simulink model "Simulink9"  (R2016b)
settings: Solver=ode4  StartTime=0.0  StopTime=30.0  FixedStep=0.005  RelTol=1e-3
values from neighbouring files (symbols this model uses):
  Kf = (1/tauf)    (= 20)    [Ejercicio9.m]
  Kt = 10/90    (= 0.111111111111)    [Ejercicio9.m]
  tauf = 1/wcf    (= 0.05)    [Ejercicio9.m]
  Vmax = 60    [Ejercicio9.m]
  wcf = 20    [Ejercicio9.m]
  wn = 20    [Ejercicio9.m]
  Xmax = 90    [Ejercicio9.m]
  zeta = 0.85    [Ejercicio9.m]
  zetaf = 1    [Ejercicio9.m]
undefined symbols (not defined in the file or in its folder): Tm
libraries: simulink x6
settings Model: Creator=elena  LastModifiedBy=elena
settings DataIOCC: ReturnWorkspaceOutputs=on
settings DebuggingCC: SFMachineParentedDataDiag=error
settings SFSimCC: SimUseLocalCustomCode=on
settings RTWCC: RTWUseLocalCustomCode=on

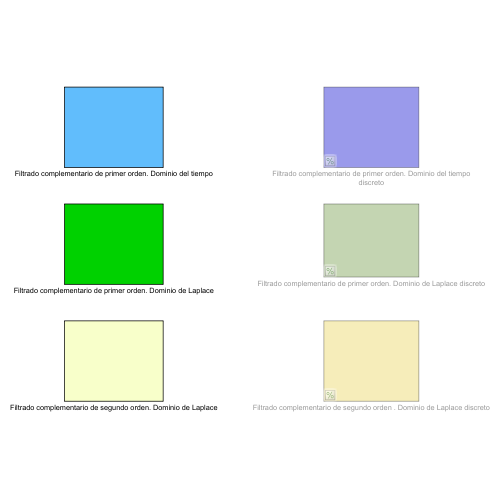
[thumbnail: Simulink's stored preview of the top-level diagram]
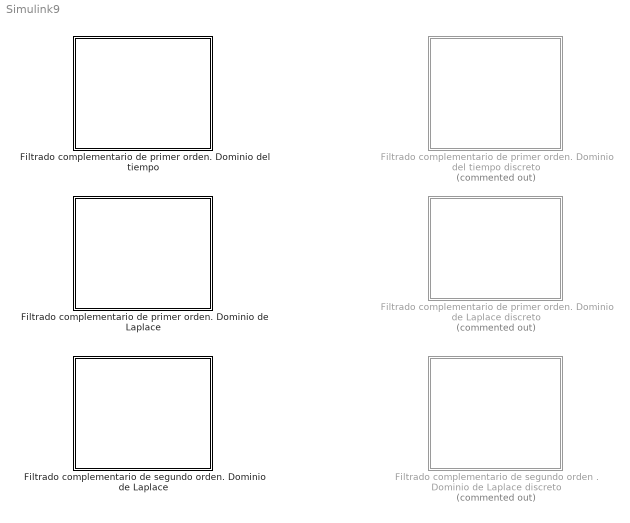
== system Simulink9 ==
  Filtrado complementario de primer orden. Dominio de Laplace : Subsystem
  Filtrado complementario de primer orden. Dominio de Laplace discreto : Subsystem  Commented=on
  "Filtrado complementario de primer orden. Dominio del tiempo " : Subsystem
  Filtrado complementario de primer orden. Dominio del tiempo discreto : Subsystem  Commented=on
  Filtrado complementario de segundo orden . Dominio de Laplace discreto : Subsystem  Commented=on
  Filtrado complementario de segundo orden. Dominio de Laplace : Subsystem

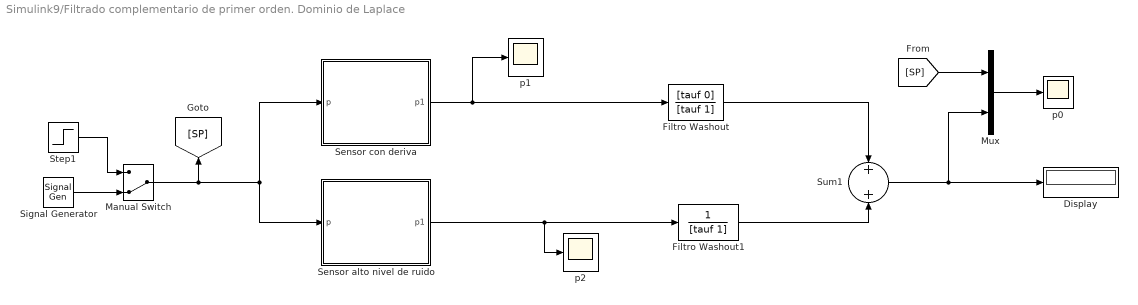
== system Simulink9/Filtrado complementario de primer orden. Dominio de Laplace ==
  Display : Display
  Filtro Washout : TransferFcn  Numerator=[tauf 0]  Denominator=[tauf 1]
  Filtro Washout1 : TransferFcn  Denominator=[tauf 1]
  Manual Switch : ManualSwitch  CurrentSetting=0
  Mux : Mux  Inputs=2
  Sensor alto nivel de ruido : Subsystem
  Sensor con deriva : Subsystem
  Signal Generator : SignalGenerator  Units=rad/sec
  Step1 : Step  SampleTime=0
  Sum1 : Sum
  p0 : Scope
  p1 : Scope
  p2 : Scope
  wires:
  Sensor alto nivel de ruido/1(p1) -> p2/1, Filtro Washout1/1
  Sensor con deriva/1(p1) -> p1/1, Filtro Washout/1
  Sum1/1 -> Mux/2, Display/1
  Filtro Washout/1 -> Sum1/1
  Filtro Washout1/1 -> Sum1/2
  Signal Generator/1 -> Manual Switch/2
  Step1/1 -> Manual Switch/1
  Manual Switch/1 -> Sensor alto nivel de ruido/1(p), Sensor con deriva/1(p), [SP]
  [SP] -> Mux/1
  Mux/1 -> p0/1

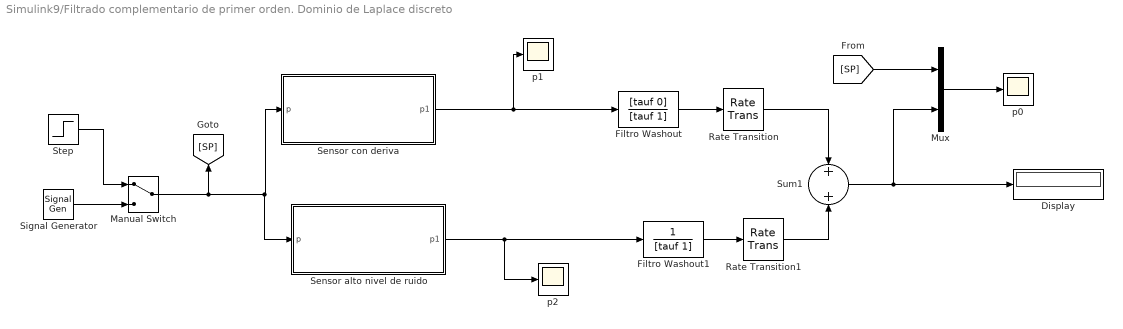
== system Simulink9/Filtrado complementario de primer orden. Dominio de Laplace discreto ==
  Display : Display
  Filtro Washout : TransferFcn  Numerator=[tauf 0]  Denominator=[tauf 1]
  Filtro Washout1 : TransferFcn  Denominator=[tauf 1]
  Manual Switch : ManualSwitch
  Mux : Mux  Inputs=2
  Rate Transition : RateTransition  OutPortSampleTime=Tm
  Rate Transition1 : RateTransition  OutPortSampleTime=Tm
  Sensor alto nivel de ruido : Subsystem
  Sensor con deriva : Subsystem
  Signal Generator : SignalGenerator  WaveForm=square  Units=rad/sec
  Step : Step  SampleTime=0
  Sum1 : Sum
  p0 : Scope
  p1 : Scope
  p2 : Scope
  wires:
  Mux/1 -> p0/1
  Sensor alto nivel de ruido/1(p1) -> Filtro Washout1/1, p2/1
  Step/1 -> Manual Switch/1
  [SP] -> Mux/1
  Manual Switch/1 -> Sensor alto nivel de ruido/1(p), Sensor con deriva/1(p), [SP]
  Sensor con deriva/1(p1) -> p1/1, Filtro Washout/1
  Sum1/1 -> Mux/2, Display/1
  Filtro Washout/1 -> Rate Transition/1
  Rate Transition/1 -> Sum1/1
  Filtro Washout1/1 -> Rate Transition1/1
  Rate Transition1/1 -> Sum1/2
  Signal Generator/1 -> Manual Switch/2

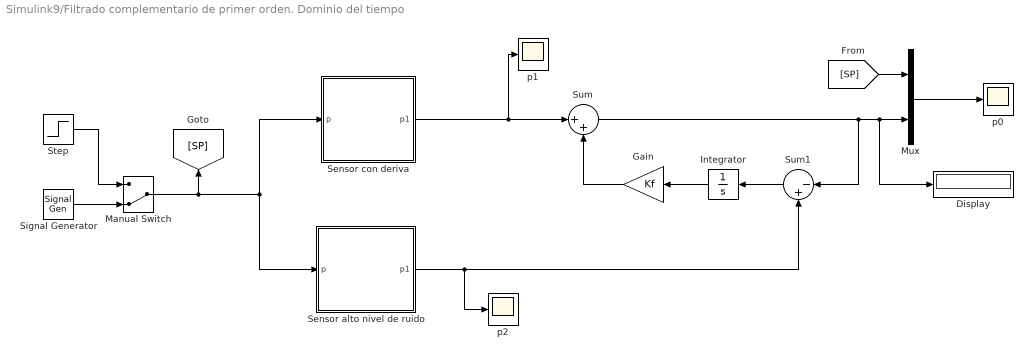
== system Simulink9/Filtrado complementario de primer orden. Dominio del tiempo  ==
  Display : Display
  Gain : Gain  Gain=Kf
  Integrator : Integrator
  Manual Switch : ManualSwitch  CurrentSetting=0
  Mux : Mux  Inputs=2
  Sensor alto nivel de ruido : Subsystem
  Sensor con deriva : Subsystem
  Signal Generator : SignalGenerator  WaveForm=square  Units=rad/sec
  Step : Step  SampleTime=0
  Sum : Sum  Inputs=|++
  Sum1 : Sum  Inputs=|-+
  p0 : Scope
  p1 : Scope
  p2 : Scope
  wires:
  Sum1/1 -> Integrator/1
  Sum/1 -> Sum1/1, Display/1, Mux/2
  Mux/1 -> p0/1
  Sensor alto nivel de ruido/1(p1) -> Sum1/2, p2/1
  Step/1 -> Manual Switch/1
  Gain/1 -> Sum/2
  [SP] -> Mux/1
  Manual Switch/1 -> Sensor alto nivel de ruido/1(p), Sensor con deriva/1(p), [SP]
  Sensor con deriva/1(p1) -> p1/1, Sum/1
  Integrator/1 -> Gain/1
  Signal Generator/1 -> Manual Switch/2

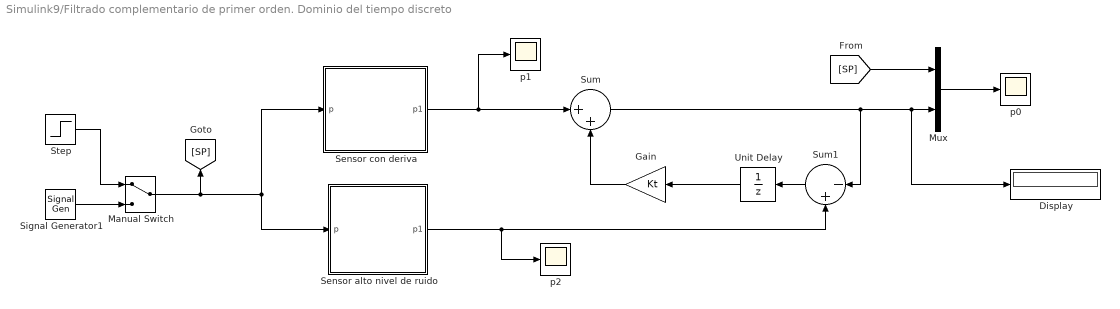
== system Simulink9/Filtrado complementario de primer orden. Dominio del tiempo discreto ==
  Display : Display
  Gain : Gain  Gain=Kt
  Manual Switch : ManualSwitch
  Mux : Mux  Inputs=2
  Sensor alto nivel de ruido : Subsystem
  Sensor con deriva : Subsystem
  Signal Generator1 : SignalGenerator  WaveForm=square  Units=rad/sec
  Step : Step  SampleTime=0
  Sum : Sum  Inputs=|++
  Sum1 : Sum  Inputs=|-+
  Unit Delay : UnitDelay  SampleTime=Tm  HasFrameUpgradeWarning=on
  p0 : Scope
  p1 : Scope
  p2 : Scope
  wires:
  Sum1/1 -> Unit Delay/1
  Sum/1 -> Display/1, Mux/2, Sum1/1
  Mux/1 -> p0/1
  Sensor alto nivel de ruido/1(p1) -> p2/1, Sum1/2
  Step/1 -> Manual Switch/1
  Gain/1 -> Sum/2
  [SP] -> Mux/1
  Manual Switch/1 -> Sensor alto nivel de ruido/1(p), Sensor con deriva/1(p), [SP]
  Sensor con deriva/1(p1) -> Sum/1, p1/1
  Unit Delay/1 -> Gain/1
  Signal Generator1/1 -> Manual Switch/2

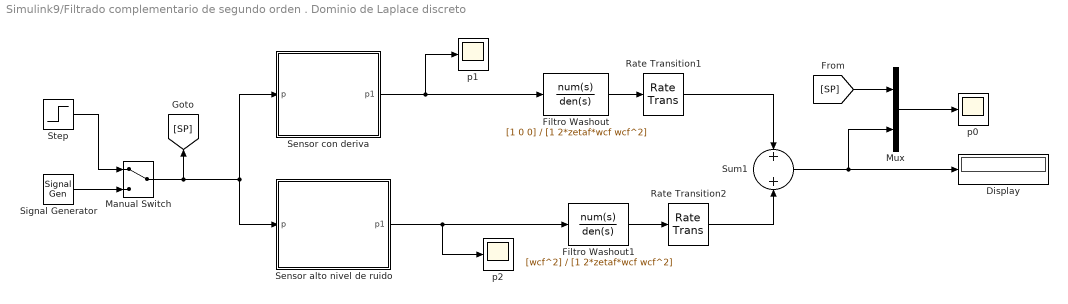
== system Simulink9/Filtrado complementario de segundo orden . Dominio de Laplace discreto ==
  Display : Display
  Filtro Washout : TransferFcn  Numerator=[1 0 0]  Denominator=[1 2*zetaf*wcf wcf^2]
  Filtro Washout1 : TransferFcn  Numerator=[wcf^2]  Denominator=[1 2*zetaf*wcf wcf^2]
  Manual Switch : ManualSwitch
  Mux : Mux  Inputs=2
  Rate Transition1 : RateTransition  OutPortSampleTime=Tm
  Rate Transition2 : RateTransition  OutPortSampleTime=Tm
  Sensor alto nivel de ruido : Subsystem
  Sensor con deriva : Subsystem
  Signal Generator : SignalGenerator  WaveForm=square  Units=rad/sec
  Step : Step  SampleTime=0
  Sum1 : Sum
  p0 : Scope
  p1 : Scope
  p2 : Scope
  wires:
  Mux/1 -> p0/1
  Sensor alto nivel de ruido/1(p1) -> p2/1, Filtro Washout1/1
  Step/1 -> Manual Switch/1
  [SP] -> Mux/1
  Manual Switch/1 -> Sensor alto nivel de ruido/1(p), Sensor con deriva/1(p), [SP]
  Sensor con deriva/1(p1) -> Filtro Washout/1, p1/1
  Sum1/1 -> Display/1, Mux/2
  Filtro Washout/1 -> Rate Transition1/1
  Rate Transition1/1 -> Sum1/1
  Filtro Washout1/1 -> Rate Transition2/1
  Rate Transition2/1 -> Sum1/2
  Signal Generator/1 -> Manual Switch/2

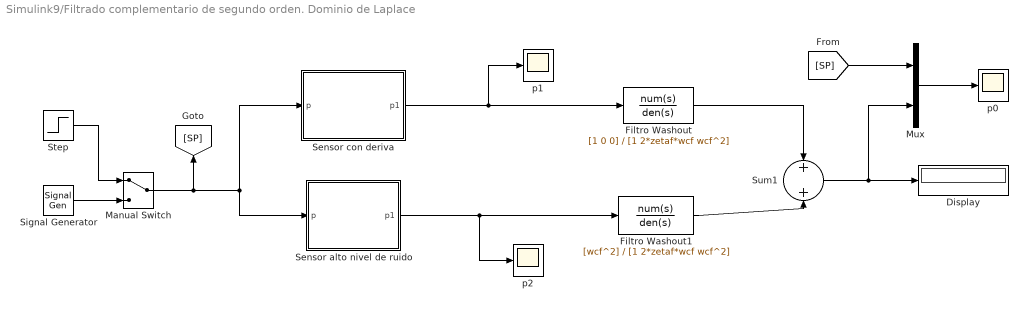
== system Simulink9/Filtrado complementario de segundo orden. Dominio de Laplace ==
  Display : Display
  Filtro Washout : TransferFcn  Numerator=[1 0 0]  Denominator=[1 2*zetaf*wcf wcf^2]
  Filtro Washout1 : TransferFcn  Numerator=[wcf^2]  Denominator=[1 2*zetaf*wcf wcf^2]
  Manual Switch : ManualSwitch
  Mux : Mux  Inputs=2
  Sensor alto nivel de ruido : Subsystem
  Sensor con deriva : Subsystem
  Signal Generator : SignalGenerator  Units=rad/sec
  Step : Step  SampleTime=0
  Sum1 : Sum
  p0 : Scope
  p1 : Scope
  p2 : Scope
  wires:
  Mux/1 -> p0/1
  Sensor alto nivel de ruido/1(p1) -> p2/1, Filtro Washout1/1
  Step/1 -> Manual Switch/1
  [SP] -> Mux/1
  Manual Switch/1 -> Sensor alto nivel de ruido/1(p), Sensor con deriva/1(p), [SP]
  Sensor con deriva/1(p1) -> p1/1, Filtro Washout/1
  Sum1/1 -> Mux/2, Display/1
  Filtro Washout/1 -> Sum1/1
  Filtro Washout1/1 -> Sum1/2
  Signal Generator/1 -> Manual Switch/2

== system Simulink9/Filtrado complementario de primer orden. Dominio de Laplace/Sensor alto nivel de ruido ==
  p : Inport
  Add : Sum
  Random Number : RandomNumber  Variance=1e-3  Seed=1234567  SampleTime=0
  dinamica del sensot : Subsystem
  p1 : Outport
  wires:
  Random Number/1 -> Add/1
  p/1 -> dinamica del sensot/1(y)
  Add/1 -> p1/1
  dinamica del sensot/1(ym) -> Add/2

== system Simulink9/Filtrado complementario de primer orden. Dominio de Laplace/Sensor con deriva ==
  p : Inport
  Add : Sum  Inputs=+++
  Ramp : simulink/Sources/Ramp  slope=0.0005  start=0  X0=0
  Random Number : RandomNumber  Variance=1e-5  Seed=1234567  SampleTime=0
  dinamica del sensot : Subsystem
  p1 : Outport
  wires:
  Ramp/1 -> Add/1
  Random Number/1 -> Add/3
  p/1 -> dinamica del sensot/1(y)
  Add/1 -> p1/1
  dinamica del sensot/1(ym) -> Add/2

== system Simulink9/Filtrado complementario de primer orden. Dominio de Laplace discreto/Sensor alto nivel de ruido ==
  p : Inport
  Add : Sum
  Random Number : RandomNumber  Variance=10^(-3)  Seed=1234567  SampleTime=0.1
  dinamica del sensot : Subsystem
  p1 : Outport
  wires:
  Random Number/1 -> Add/1
  p/1 -> dinamica del sensot/1(y)
  Add/1 -> p1/1
  dinamica del sensot/1(ym) -> Add/2

== system Simulink9/Filtrado complementario de primer orden. Dominio de Laplace discreto/Sensor con deriva ==
  p : Inport
  Add : Sum  Inputs=+++
  Ramp : simulink/Sources/Ramp  slope=0.0005  start=0  X0=0
  Random Number : RandomNumber  Variance=10^(-5)  Seed=1234567  SampleTime=0.1
  dinamica del sensot : Subsystem
  p1 : Outport
  wires:
  Ramp/1 -> Add/1
  Random Number/1 -> Add/3
  p/1 -> dinamica del sensot/1(y)
  Add/1 -> p1/1
  dinamica del sensot/1(ym) -> Add/2

== system Simulink9/Filtrado complementario de primer orden. Dominio del tiempo /Sensor alto nivel de ruido ==
  p : Inport
  Add : Sum
  Random Number : RandomNumber  Variance=1e-3  Seed=1234567  SampleTime=0
  dinamica del sensot : Subsystem
  p1 : Outport
  wires:
  Random Number/1 -> Add/1
  p/1 -> dinamica del sensot/1(y)
  Add/1 -> p1/1
  dinamica del sensot/1(ym) -> Add/2

== system Simulink9/Filtrado complementario de primer orden. Dominio del tiempo /Sensor con deriva ==
  p : Inport
  Add : Sum  Inputs=+++
  Ramp : simulink/Sources/Ramp  slope=0.0005  start=0  X0=0
  Random Number : RandomNumber  Variance=1e-5  Seed=1234567  SampleTime=0
  dinamica del sensor : Subsystem
  p1 : Outport
  wires:
  Ramp/1 -> Add/1
  Random Number/1 -> Add/3
  p/1 -> dinamica del sensor/1(y)
  Add/1 -> p1/1
  dinamica del sensor/1(ym) -> Add/2

== system Simulink9/Filtrado complementario de primer orden. Dominio del tiempo discreto/Sensor alto nivel de ruido ==
  p : Inport
  Add : Sum
  Random Number : RandomNumber  Variance=10^(-3)  Seed=1234567  SampleTime=0.1
  dinamica del sensot : Subsystem
  p1 : Outport
  wires:
  Random Number/1 -> Add/1
  p/1 -> dinamica del sensot/1(y)
  Add/1 -> p1/1
  dinamica del sensot/1(ym) -> Add/2

== system Simulink9/Filtrado complementario de primer orden. Dominio del tiempo discreto/Sensor con deriva ==
  p : Inport
  Add : Sum  Inputs=+++
  Ramp : simulink/Sources/Ramp  slope=0.0005  start=0  X0=0
  Random Number : RandomNumber  Variance=10^(-5)  Seed=1234567  SampleTime=0.1
  dinamica del sensot : Subsystem
  p1 : Outport
  wires:
  Ramp/1 -> Add/1
  Random Number/1 -> Add/3
  p/1 -> dinamica del sensot/1(y)
  Add/1 -> p1/1
  dinamica del sensot/1(ym) -> Add/2

== system Simulink9/Filtrado complementario de segundo orden . Dominio de Laplace discreto/Sensor alto nivel de ruido ==
  p : Inport
  Add : Sum
  Random Number : RandomNumber  Variance=10^(-3)  Seed=1234567  SampleTime=0.1
  dinamica del sensot : Subsystem
  p1 : Outport
  wires:
  Random Number/1 -> Add/1
  p/1 -> dinamica del sensot/1(y)
  Add/1 -> p1/1
  dinamica del sensot/1(ym) -> Add/2

== system Simulink9/Filtrado complementario de segundo orden . Dominio de Laplace discreto/Sensor con deriva ==
  p : Inport
  Add : Sum  Inputs=+++
  Ramp : simulink/Sources/Ramp  slope=0.0005  start=0  X0=0
  Random Number : RandomNumber  Variance=10^(-5)  Seed=1234567  SampleTime=0.1
  dinamica del sensot : Subsystem
  p1 : Outport
  wires:
  Ramp/1 -> Add/1
  Random Number/1 -> Add/3
  p/1 -> dinamica del sensot/1(y)
  Add/1 -> p1/1
  dinamica del sensot/1(ym) -> Add/2

== system Simulink9/Filtrado complementario de segundo orden. Dominio de Laplace/Sensor alto nivel de ruido ==
  p : Inport
  Add : Sum
  Random Number : RandomNumber  Variance=10^(-3)  Seed=1234567  SampleTime=0.1
  dinamica del sensot : Subsystem
  p1 : Outport
  wires:
  Random Number/1 -> Add/1
  p/1 -> dinamica del sensot/1(y)
  Add/1 -> p1/1
  dinamica del sensot/1(ym) -> Add/2

== system Simulink9/Filtrado complementario de segundo orden. Dominio de Laplace/Sensor con deriva ==
  p : Inport
  Add : Sum  Inputs=+++
  Ramp : simulink/Sources/Ramp  slope=0.0005  start=0  X0=0
  Random Number : RandomNumber  Variance=10^(-5)  Seed=1234567  SampleTime=0.1
  dinamica del sensot : Subsystem
  p1 : Outport
  wires:
  Ramp/1 -> Add/1
  Random Number/1 -> Add/3
  p/1 -> dinamica del sensot/1(y)
  Add/1 -> p1/1
  dinamica del sensot/1(ym) -> Add/2

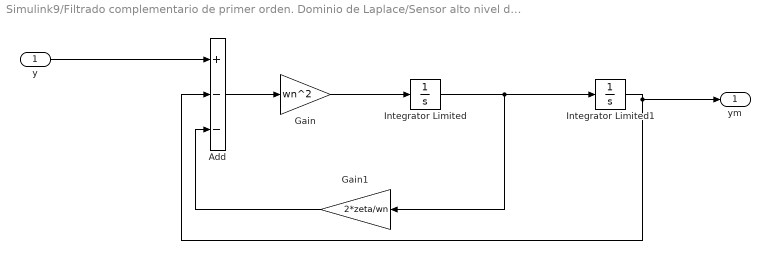
== system Simulink9/Filtrado complementario de primer orden. Dominio de Laplace/Sensor alto nivel de ruido/dinamica del sensot ==
  y : Inport
  Add : Sum  Inputs=+--
  Gain : Gain  Gain=wn^2
  Gain1 : Gain  Gain=2*zeta/wn
  Integrator Limited : Integrator  LimitOutput=on  UpperSaturationLimit=Vmax  LowerSaturationLimit=-Vmax
  Integrator Limited1 : Integrator  LimitOutput=on  UpperSaturationLimit=Xmax  LowerSaturationLimit=-Xmax
  ym : Outport
  wires:
  Gain/1 -> Integrator Limited/1
  Gain1/1 -> Add/3
  y/1 -> Add/1
  Integrator Limited1/1 -> ym/1, Add/2
  Integrator Limited/1 -> Gain1/1, Integrator Limited1/1
  Add/1 -> Gain/1

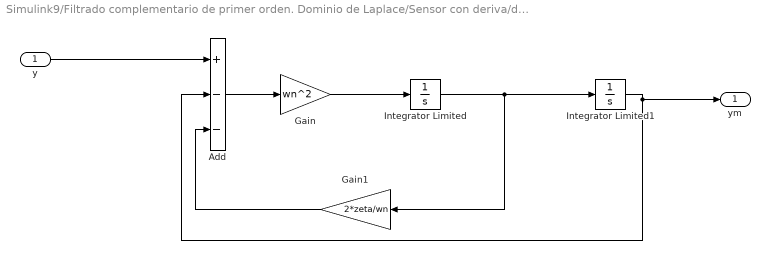
== system Simulink9/Filtrado complementario de primer orden. Dominio de Laplace/Sensor con deriva/dinamica del sensot ==
  y : Inport
  Add : Sum  Inputs=+--
  Gain : Gain  Gain=wn^2
  Gain1 : Gain  Gain=2*zeta/wn
  Integrator Limited : Integrator  LimitOutput=on  UpperSaturationLimit=Vmax  LowerSaturationLimit=-Vmax
  Integrator Limited1 : Integrator  LimitOutput=on  UpperSaturationLimit=Xmax  LowerSaturationLimit=-Xmax
  ym : Outport
  wires:
  Gain/1 -> Integrator Limited/1
  Gain1/1 -> Add/3
  y/1 -> Add/1
  Integrator Limited1/1 -> ym/1, Add/2
  Integrator Limited/1 -> Gain1/1, Integrator Limited1/1
  Add/1 -> Gain/1

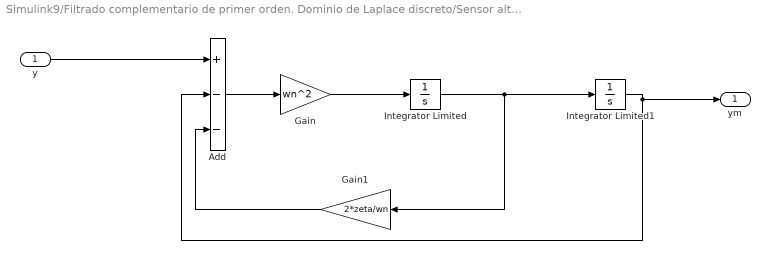
== system Simulink9/Filtrado complementario de primer orden. Dominio de Laplace discreto/Sensor alto nivel de ruido/dinamica del sensot ==
  y : Inport
  Add : Sum  Inputs=+--
  Gain : Gain  Gain=wn^2
  Gain1 : Gain  Gain=2*zeta/wn
  Integrator Limited : Integrator  LimitOutput=on  UpperSaturationLimit=Vmax  LowerSaturationLimit=-Vmax
  Integrator Limited1 : Integrator  LimitOutput=on  UpperSaturationLimit=Xmax  LowerSaturationLimit=-Xmax
  ym : Outport
  wires:
  Gain/1 -> Integrator Limited/1
  Gain1/1 -> Add/3
  y/1 -> Add/1
  Integrator Limited1/1 -> ym/1, Add/2
  Integrator Limited/1 -> Gain1/1, Integrator Limited1/1
  Add/1 -> Gain/1

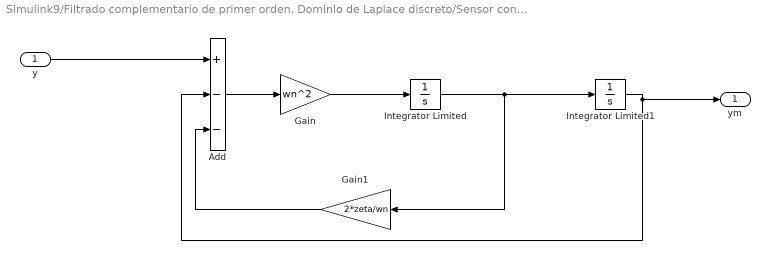
== system Simulink9/Filtrado complementario de primer orden. Dominio de Laplace discreto/Sensor con deriva/dinamica del sensot ==
  y : Inport
  Add : Sum  Inputs=+--
  Gain : Gain  Gain=wn^2
  Gain1 : Gain  Gain=2*zeta/wn
  Integrator Limited : Integrator  LimitOutput=on  UpperSaturationLimit=Vmax  LowerSaturationLimit=-Vmax
  Integrator Limited1 : Integrator  LimitOutput=on  UpperSaturationLimit=Xmax  LowerSaturationLimit=-Xmax
  ym : Outport
  wires:
  Gain/1 -> Integrator Limited/1
  Gain1/1 -> Add/3
  y/1 -> Add/1
  Integrator Limited1/1 -> ym/1, Add/2
  Integrator Limited/1 -> Gain1/1, Integrator Limited1/1
  Add/1 -> Gain/1

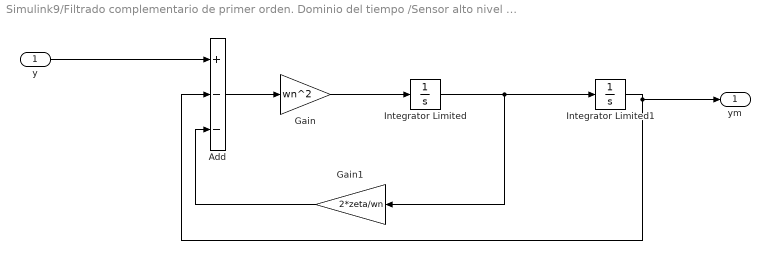
== system Simulink9/Filtrado complementario de primer orden. Dominio del tiempo /Sensor alto nivel de ruido/dinamica del sensot ==
  y : Inport
  Add : Sum  Inputs=+--
  Gain : Gain  Gain=wn^2
  Gain1 : Gain  Gain=2*zeta/wn
  Integrator Limited : Integrator  LimitOutput=on  UpperSaturationLimit=Vmax  LowerSaturationLimit=-Vmax
  Integrator Limited1 : Integrator  LimitOutput=on  UpperSaturationLimit=Xmax  LowerSaturationLimit=-Xmax
  ym : Outport
  wires:
  Gain/1 -> Integrator Limited/1
  Gain1/1 -> Add/3
  y/1 -> Add/1
  Integrator Limited1/1 -> ym/1, Add/2
  Integrator Limited/1 -> Integrator Limited1/1, Gain1/1
  Add/1 -> Gain/1

== system Simulink9/Filtrado complementario de primer orden. Dominio del tiempo /Sensor con deriva/dinamica del sensor ==
  y : Inport
  Add : Sum  Inputs=+--
  Gain : Gain  Gain=wn^2
  Gain1 : Gain  Gain=2*zeta/wn
  Integrator Limited : Integrator  LimitOutput=on  UpperSaturationLimit=Vmax  LowerSaturationLimit=-Vmax
  Integrator Limited1 : Integrator  LimitOutput=on  UpperSaturationLimit=Xmax  LowerSaturationLimit=-Xmax
  ym : Outport
  wires:
  Gain/1 -> Integrator Limited/1
  Gain1/1 -> Add/3
  y/1 -> Add/1
  Integrator Limited1/1 -> Add/2, ym/1
  Integrator Limited/1 -> Gain1/1, Integrator Limited1/1
  Add/1 -> Gain/1

== system Simulink9/Filtrado complementario de primer orden. Dominio del tiempo discreto/Sensor alto nivel de ruido/dinamica del sensot ==
  y : Inport
  Add : Sum  Inputs=+--
  Gain : Gain  Gain=wn^2
  Gain1 : Gain  Gain=2*zeta/wn
  Integrator Limited : Integrator  LimitOutput=on  UpperSaturationLimit=Vmax  LowerSaturationLimit=-Vmax
  Integrator Limited1 : Integrator  LimitOutput=on  UpperSaturationLimit=Xmax  LowerSaturationLimit=-Xmax
  ym : Outport
  wires:
  Gain/1 -> Integrator Limited/1
  Gain1/1 -> Add/3
  y/1 -> Add/1
  Integrator Limited1/1 -> ym/1, Add/2
  Integrator Limited/1 -> Integrator Limited1/1, Gain1/1
  Add/1 -> Gain/1

== system Simulink9/Filtrado complementario de primer orden. Dominio del tiempo discreto/Sensor con deriva/dinamica del sensot ==
  y : Inport
  Add : Sum  Inputs=+--
  Gain : Gain  Gain=wn^2
  Gain1 : Gain  Gain=2*zeta/wn
  Integrator Limited : Integrator  LimitOutput=on  UpperSaturationLimit=Vmax  LowerSaturationLimit=-Vmax
  Integrator Limited1 : Integrator  LimitOutput=on  UpperSaturationLimit=Xmax  LowerSaturationLimit=-Xmax
  ym : Outport
  wires:
  Gain/1 -> Integrator Limited/1
  Gain1/1 -> Add/3
  y/1 -> Add/1
  Integrator Limited1/1 -> ym/1, Add/2
  Integrator Limited/1 -> Gain1/1, Integrator Limited1/1
  Add/1 -> Gain/1

== system Simulink9/Filtrado complementario de segundo orden . Dominio de Laplace discreto/Sensor alto nivel de ruido/dinamica del sensot ==
  y : Inport
  Add : Sum  Inputs=+--
  Gain : Gain  Gain=wn^2
  Gain1 : Gain  Gain=2*zeta/wn
  Integrator Limited : Integrator  LimitOutput=on  UpperSaturationLimit=Vmax  LowerSaturationLimit=-Vmax
  Integrator Limited1 : Integrator  LimitOutput=on  UpperSaturationLimit=Xmax  LowerSaturationLimit=-Xmax
  ym : Outport
  wires:
  Gain/1 -> Integrator Limited/1
  Gain1/1 -> Add/3
  y/1 -> Add/1
  Integrator Limited1/1 -> ym/1, Add/2
  Integrator Limited/1 -> Gain1/1, Integrator Limited1/1
  Add/1 -> Gain/1

== system Simulink9/Filtrado complementario de segundo orden . Dominio de Laplace discreto/Sensor con deriva/dinamica del sensot ==
  y : Inport
  Add : Sum  Inputs=+--
  Gain : Gain  Gain=wn^2
  Gain1 : Gain  Gain=2*zeta/wn
  Integrator Limited : Integrator  LimitOutput=on  UpperSaturationLimit=Vmax  LowerSaturationLimit=-Vmax
  Integrator Limited1 : Integrator  LimitOutput=on  UpperSaturationLimit=Xmax  LowerSaturationLimit=-Xmax
  ym : Outport
  wires:
  Gain/1 -> Integrator Limited/1
  Gain1/1 -> Add/3
  y/1 -> Add/1
  Integrator Limited1/1 -> ym/1, Add/2
  Integrator Limited/1 -> Gain1/1, Integrator Limited1/1
  Add/1 -> Gain/1

== system Simulink9/Filtrado complementario de segundo orden. Dominio de Laplace/Sensor alto nivel de ruido/dinamica del sensot ==
  y : Inport
  Add : Sum  Inputs=+--
  Gain : Gain  Gain=wn^2
  Gain1 : Gain  Gain=2*zeta/wn
  Integrator Limited : Integrator  LimitOutput=on  UpperSaturationLimit=Vmax  LowerSaturationLimit=-Vmax
  Integrator Limited1 : Integrator  LimitOutput=on  UpperSaturationLimit=Xmax  LowerSaturationLimit=-Xmax
  ym : Outport
  wires:
  Gain/1 -> Integrator Limited/1
  Gain1/1 -> Add/3
  y/1 -> Add/1
  Integrator Limited1/1 -> ym/1, Add/2
  Integrator Limited/1 -> Gain1/1, Integrator Limited1/1
  Add/1 -> Gain/1

== system Simulink9/Filtrado complementario de segundo orden. Dominio de Laplace/Sensor con deriva/dinamica del sensot ==
  y : Inport
  Add : Sum  Inputs=+--
  Gain : Gain  Gain=wn^2
  Gain1 : Gain  Gain=2*zeta/wn
  Integrator Limited : Integrator  LimitOutput=on  UpperSaturationLimit=Vmax  LowerSaturationLimit=-Vmax
  Integrator Limited1 : Integrator  LimitOutput=on  UpperSaturationLimit=Xmax  LowerSaturationLimit=-Xmax
  ym : Outport
  wires:
  Gain/1 -> Integrator Limited/1
  Gain1/1 -> Add/3
  y/1 -> Add/1
  Integrator Limited1/1 -> ym/1, Add/2
  Integrator Limited/1 -> Gain1/1, Integrator Limited1/1
  Add/1 -> Gain/1
